simulink model "FSAC2021_V1_Running"  (R2014a)
settings: Solver=FixedStepDiscrete  StartTime=0.0  StopTime=inf  FixedStep=0.0005  RelTol=1e-3
model workspace (MAT data in the model file):
  MCOS : class17 (value not decoded)
  MCOS : class17 (value not decoded)
  MCOS : class17 (value not decoded)
  MCOS : class17 (value not decoded)
  MCOS : class17 (value not decoded)
  MCOS : class17 (value not decoded)
  MCOS : class17 (value not decoded)
  MCOS : class17 (value not decoded)
  MCOS : class17 (value not decoded)
  MCOS : class17 (value not decoded)
  MCOS : class17 (value not decoded)
  MCOS : class17 (value not decoded)
  MCOS : class17 (value not decoded)
  MCOS : class17 (value not decoded)
  MCOS : class17 (value not decoded)
  MCOS : class17 (value not decoded)
  MCOS : class17 (value not decoded)
  MCOS : class17 (value not decoded)
  MCOS : class17 (value not decoded)
  BUZZER_START = 1
  MCOS : class17 (value not decoded)
  MCOS : class17 (value not decoded)
  MCOS : class17 (value not decoded)
  MCOS : class17 (value not decoded)
  MCOS : class17 (value not decoded)
  MCOS : class17 (value not decoded)
  MCOS : class17 (value not decoded)
  MCOS : class17 (value not decoded)
  MCOS : class17 (value not decoded)
  MCOS : class17 (value not decoded)
  MCOS : class17 (value not decoded)
  MCOS : class17 (value not decoded)
  MCOS : class17 (value not decoded)
  MCOS : class17 (value not decoded)
  MCOS : class17 (value not decoded)
  MCOS : class17 (value not decoded)
  MCOS : class17 (value not decoded)
  MCOS : class17 (value not decoded)
  MCOS : class17 (value not decoded)
  MCOS : class17 (value not decoded)
  MCOS : class17 (value not decoded)
  MCOS : class17 (value not decoded)
  MCOS : class17 (value not decoded)
  MCOS : class17 (value not decoded)
  MCOS : class17 (value not decoded)
  MCOS : class17 (value not decoded)
  MCOS : class17 (value not decoded)
  MCOS : class17 (value not decoded)
  MCOS : class17 (value not decoded)
  MCOS : class17 (value not decoded)
  MCOS : class17 (value not decoded)
  MCOS : class17 (value not decoded)
  MCOS : class17 (value not decoded)
  MCOS : class17 (value not decoded)
  MCOS : class17 (value not decoded)
  MCOS : class17 (value not decoded)
  MCOS : class17 (value not decoded)
  MCOS : class17 (value not decoded)
  Brake = 11
  MCOS : class17 (value not decoded)
  MCOS : class17 (value not decoded)
  MCOS : class17 (value not decoded)
  MCOS : class17 (value not decoded)
  MCOS : class17 (value not decoded)
  MCOS : class17 (value not decoded)
  MCOS : class17 (value not decoded)
  MCOS : class17 (value not decoded)
  Sensor_Acc_b = 101.85
  Sensor_Acc_k = -0.0185
  Str_Sen_Orig_Angle = -341
  MCOS : class17 (value not decoded)
  Tire_D = 0.47
  T = 0.05
libraries: simulink x402, ec55xxlib x134
(part 9 of 17)

== system FSAC2021_V1_Running/ROUTING/TO_ACAN/DV_driving_dynamics_2/Acceleration_longitudinal ==
  Acceleration_longitudinal : Inport
  Acceleration_longitudinalABS : Abs
  Acceleration_longitudinalCOV : DataTypeConversion  OutDataTypeStr=uint8
  Acceleration_longitudinalCS : ArithShift  BitShiftNumber=-16
  Acceleration_longitudinalConS : Constant  OutDataTypeStr=single
  Acceleration_longitudinalCosR : Constant  Value=0  OutDataTypeStr=uint8
  Acceleration_longitudinalROP : RelationalOperator  Operator=<  OutDataTypeStr=boolean
  Acceleration_longitudinalRon : Rounding  Operator=round
  Acceleration_longitudinalSW : Switch  Criteria=u2 ~= 0
  Acceleration_longitudinal_1sat : Saturate  UpperLimit=65535  LowerLimit=0
  Acceleration_longitudinal_And : simulink/Logic and Bit Operations/Bitwise Operator  logicop=AND  UseBitMask=off  NumInputPorts=2  BitMask=bin2dec('11011001')  BitMaskRealWorld=Stored Integer
  Acceleration_longitudinal_And_C : Constant  Value=255  OutDataTypeStr=uint32
  Acceleration_longitudinal_Convert : DataTypeConversion  OutDataTypeStr=uint32
  Acceleration_longitudinal_D : Product  Inputs=*/
  Acceleration_longitudinal_D1 : Product  Inputs=*/
  Acceleration_longitudinal_F : Constant  Value=0.001953125  OutDataTypeStr=single
  Acceleration_longitudinal_L : simulink/Logic and Bit Operations/Bitwise Operator  logicop=AND  UseBitMask=on  BitMask=65535  BitMaskRealWorld=Stored Integer
  Acceleration_longitudinal_O : Constant  Value=0  OutDataTypeStr=single
  Acceleration_longitudinal_S : ArithShift
  Acceleration_longitudinal_sat : Saturate  UpperLimit=63.998046875  LowerLimit=-64
  Acceleration_longitudinal_st : Sum  Inputs=+-
  Acceleration_longitudinaloutput2_C : Constant  Value=256
  Acceleration_longitudinalsubcon : Sum  Inputs=+-
  BitCov : DataTypeConversion  OutDataTypeStr=uint8
  output1 : Outport
  output2 : Outport  Port=2
  wires:
  Acceleration_longitudinal/1 -> Acceleration_longitudinal_sat/1
  Acceleration_longitudinal_sat/1 -> Acceleration_longitudinal_st/1
  Acceleration_longitudinal_O/1 -> Acceleration_longitudinal_st/2
  Acceleration_longitudinal_st/1 -> Acceleration_longitudinal_D/1
  Acceleration_longitudinal_F/1 -> Acceleration_longitudinal_D/2
  Acceleration_longitudinal_D/1 -> Acceleration_longitudinalRon/1
  Acceleration_longitudinalRon/1 -> Acceleration_longitudinalROP/1, Acceleration_longitudinalABS/1, Acceleration_longitudinalSW/3
  Acceleration_longitudinalCosR/1 -> Acceleration_longitudinalROP/2
  Acceleration_longitudinalConS/1 -> Acceleration_longitudinalCS/1
  Acceleration_longitudinalCS/1 -> Acceleration_longitudinalsubcon/1
  Acceleration_longitudinalABS/1 -> Acceleration_longitudinalsubcon/2
  Acceleration_longitudinalsubcon/1 -> Acceleration_longitudinalSW/1
  Acceleration_longitudinalROP/1 -> Acceleration_longitudinalSW/2
  Acceleration_longitudinalSW/1 -> Acceleration_longitudinal_S/1
  Acceleration_longitudinal_S/1 -> Acceleration_longitudinal_1sat/1
  Acceleration_longitudinal_1sat/1 -> Acceleration_longitudinal_Convert/1
  Acceleration_longitudinal_Convert/1 -> Acceleration_longitudinal_L/1
  Acceleration_longitudinal_L/1 -> Acceleration_longitudinal_D1/1, Acceleration_longitudinal_And/1
  Acceleration_longitudinaloutput2_C/1 -> Acceleration_longitudinal_D1/2
  Acceleration_longitudinal_D1/1 -> Acceleration_longitudinalCOV/1
  Acceleration_longitudinalCOV/1 -> output2/1
  Acceleration_longitudinal_And_C/1 -> Acceleration_longitudinal_And/2
  Acceleration_longitudinal_And/1 -> BitCov/1
  BitCov/1 -> output1/1

== system FSAC2021_V1_Running/ROUTING/TO_ACAN/DV_driving_dynamics_2/Yaw_rate ==
  Yaw_rate : Inport
  BitCov : DataTypeConversion  OutDataTypeStr=uint8
  Yaw_rateABS : Abs
  Yaw_rateCOV : DataTypeConversion  OutDataTypeStr=uint8
  Yaw_rateCS : ArithShift  BitShiftNumber=-16
  Yaw_rateConS : Constant  OutDataTypeStr=single
  Yaw_rateCosR : Constant  Value=0  OutDataTypeStr=uint8
  Yaw_rateROP : RelationalOperator  Operator=<  OutDataTypeStr=boolean
  Yaw_rateRon : Rounding  Operator=round
  Yaw_rateSW : Switch  Criteria=u2 ~= 0
  Yaw_rate_1sat : Saturate  UpperLimit=65535  LowerLimit=0
  Yaw_rate_And : simulink/Logic and Bit Operations/Bitwise Operator  logicop=AND  UseBitMask=off  NumInputPorts=2  BitMask=bin2dec('11011001')  BitMaskRealWorld=Stored Integer
  Yaw_rate_And_C : Constant  Value=255  OutDataTypeStr=uint32
  Yaw_rate_Convert : DataTypeConversion  OutDataTypeStr=uint32
  Yaw_rate_D : Product  Inputs=*/
  Yaw_rate_D1 : Product  Inputs=*/
  Yaw_rate_F : Constant  Value=0.0078125  OutDataTypeStr=single
  Yaw_rate_L : simulink/Logic and Bit Operations/Bitwise Operator  logicop=AND  UseBitMask=on  BitMask=65535  BitMaskRealWorld=Stored Integer
  Yaw_rate_O : Constant  Value=0  OutDataTypeStr=single
  Yaw_rate_S : ArithShift
  Yaw_rate_sat : Saturate  UpperLimit=255.9921875  LowerLimit=-256
  Yaw_rate_st : Sum  Inputs=+-
  Yaw_rateoutput4_C : Constant  Value=256
  Yaw_ratesubcon : Sum  Inputs=+-
  output3 : Outport
  output4 : Outport  Port=2
  wires:
  Yaw_rate/1 -> Yaw_rate_sat/1
  Yaw_rate_sat/1 -> Yaw_rate_st/1
  Yaw_rate_O/1 -> Yaw_rate_st/2
  Yaw_rate_st/1 -> Yaw_rate_D/1
  Yaw_rate_F/1 -> Yaw_rate_D/2
  Yaw_rate_D/1 -> Yaw_rateRon/1
  Yaw_rateRon/1 -> Yaw_rateROP/1, Yaw_rateABS/1, Yaw_rateSW/3
  Yaw_rateCosR/1 -> Yaw_rateROP/2
  Yaw_rateConS/1 -> Yaw_rateCS/1
  Yaw_rateCS/1 -> Yaw_ratesubcon/1
  Yaw_rateABS/1 -> Yaw_ratesubcon/2
  Yaw_ratesubcon/1 -> Yaw_rateSW/1
  Yaw_rateROP/1 -> Yaw_rateSW/2
  Yaw_rateSW/1 -> Yaw_rate_S/1
  Yaw_rate_S/1 -> Yaw_rate_1sat/1
  Yaw_rate_1sat/1 -> Yaw_rate_Convert/1
  Yaw_rate_Convert/1 -> Yaw_rate_L/1
  Yaw_rate_L/1 -> Yaw_rate_D1/1, Yaw_rate_And/1
  Yaw_rateoutput4_C/1 -> Yaw_rate_D1/2
  Yaw_rate_D1/1 -> Yaw_rateCOV/1
  Yaw_rateCOV/1 -> output4/1
  Yaw_rate_And_C/1 -> Yaw_rate_And/2
  Yaw_rate_And/1 -> BitCov/1
  BitCov/1 -> output3/1

== system FSAC2021_V1_Running/ROUTING/TO_ACAN/DV_system_status/AMI_State ==
  AMI_State : Inport
  AMI_StateRon : Rounding  Operator=round
  AMI_State_1sat : Saturate  UpperLimit=7  LowerLimit=0
  AMI_State_Convert : DataTypeConversion  OutDataTypeStr=uint8
  AMI_State_Convert1 : DataTypeConversion  OutDataTypeStr=uint32
  AMI_State_D : Product  Inputs=*/
  AMI_State_F : Constant  OutDataTypeStr=single
  AMI_State_L : simulink/Logic and Bit Operations/Bitwise Operator  logicop=AND  UseBitMask=on  BitMask=7  BitMaskRealWorld=Stored Integer
  AMI_State_O : Constant  Value=0  OutDataTypeStr=single
  AMI_State_S : ArithShift
  AMI_State_sat : Saturate  UpperLimit=5  LowerLimit=0
  AMI_State_st : Sum  Inputs=+-
  output1 : Outport
  wires:
  AMI_State/1 -> AMI_State_sat/1
  AMI_State_sat/1 -> AMI_State_st/1
  AMI_State_O/1 -> AMI_State_st/2
  AMI_State_st/1 -> AMI_State_D/1
  AMI_State_F/1 -> AMI_State_D/2
  AMI_State_D/1 -> AMI_StateRon/1
  AMI_StateRon/1 -> AMI_State_S/1
  AMI_State_S/1 -> AMI_State_1sat/1
  AMI_State_1sat/1 -> AMI_State_Convert1/1
  AMI_State_Convert1/1 -> AMI_State_L/1
  AMI_State_L/1 -> AMI_State_Convert/1
  AMI_State_Convert/1 -> output1/1

== system FSAC2021_V1_Running/ROUTING/TO_ACAN/DV_system_status/ASSI_State ==
  ASSI_State : Inport
  ASSI_StateRon : Rounding  Operator=round
  ASSI_State_1sat : Saturate  UpperLimit=56  LowerLimit=0
  ASSI_State_Convert : DataTypeConversion  OutDataTypeStr=uint8
  ASSI_State_Convert1 : DataTypeConversion  OutDataTypeStr=uint32
  ASSI_State_D : Product  Inputs=*/
  ASSI_State_F : Constant  OutDataTypeStr=single
  ASSI_State_L : simulink/Logic and Bit Operations/Bitwise Operator  logicop=AND  UseBitMask=on  BitMask=56  BitMaskRealWorld=Stored Integer
  ASSI_State_O : Constant  Value=0  OutDataTypeStr=single
  ASSI_State_S : ArithShift  BitShiftNumber=-3
  ASSI_State_sat : Saturate  UpperLimit=6  LowerLimit=1
  ASSI_State_st : Sum  Inputs=+-
  output1 : Outport
  wires:
  ASSI_State/1 -> ASSI_State_sat/1
  ASSI_State_sat/1 -> ASSI_State_st/1
  ASSI_State_O/1 -> ASSI_State_st/2
  ASSI_State_st/1 -> ASSI_State_D/1
  ASSI_State_F/1 -> ASSI_State_D/2
  ASSI_State_D/1 -> ASSI_StateRon/1
  ASSI_StateRon/1 -> ASSI_State_S/1
  ASSI_State_S/1 -> ASSI_State_1sat/1
  ASSI_State_1sat/1 -> ASSI_State_Convert1/1
  ASSI_State_Convert1/1 -> ASSI_State_L/1
  ASSI_State_L/1 -> ASSI_State_Convert/1
  ASSI_State_Convert/1 -> output1/1

== system FSAC2021_V1_Running/ROUTING/TO_ACAN/DV_system_status/Cones_count_actual ==
  Cones_count_actual : Inport
  BitCov : DataTypeConversion  OutDataTypeStr=uint8
  Cones_count_actualCOV : DataTypeConversion  OutDataTypeStr=uint8
  Cones_count_actualRon : Rounding  Operator=round
  Cones_count_actual_1sat : Saturate  UpperLimit=32640  LowerLimit=0
  Cones_count_actual_And : simulink/Logic and Bit Operations/Bitwise Operator  logicop=AND  UseBitMask=off  NumInputPorts=2  BitMask=bin2dec('11011001')  BitMaskRealWorld=Stored Integer
  Cones_count_actual_And_C : Constant  Value=255  OutDataTypeStr=uint32
  Cones_count_actual_Convert : DataTypeConversion  OutDataTypeStr=uint32
  Cones_count_actual_D : Product  Inputs=*/
  Cones_count_actual_D1 : Product  Inputs=*/
  Cones_count_actual_F : Constant  OutDataTypeStr=single
  Cones_count_actual_L : simulink/Logic and Bit Operations/Bitwise Operator  logicop=AND  UseBitMask=on  BitMask=32640  BitMaskRealWorld=Stored Integer
  Cones_count_actual_O : Constant  Value=0  OutDataTypeStr=single
  Cones_count_actual_S : ArithShift  BitShiftNumber=-7
  Cones_count_actual_sat : Saturate  UpperLimit=255  LowerLimit=0
  Cones_count_actual_st : Sum  Inputs=+-
  Cones_count_actualoutput3_C : Constant  Value=256
  output2 : Outport
  output3 : Outport  Port=2
  wires:
  Cones_count_actual/1 -> Cones_count_actual_sat/1
  Cones_count_actual_sat/1 -> Cones_count_actual_st/1
  Cones_count_actual_O/1 -> Cones_count_actual_st/2
  Cones_count_actual_st/1 -> Cones_count_actual_D/1
  Cones_count_actual_F/1 -> Cones_count_actual_D/2
  Cones_count_actual_D/1 -> Cones_count_actualRon/1
  Cones_count_actualRon/1 -> Cones_count_actual_S/1
  Cones_count_actual_S/1 -> Cones_count_actual_1sat/1
  Cones_count_actual_1sat/1 -> Cones_count_actual_Convert/1
  Cones_count_actual_Convert/1 -> Cones_count_actual_L/1
  Cones_count_actual_L/1 -> Cones_count_actual_D1/1, Cones_count_actual_And/1
  Cones_count_actualoutput3_C/1 -> Cones_count_actual_D1/2
  Cones_count_actual_D1/1 -> Cones_count_actualCOV/1
  Cones_count_actualCOV/1 -> output3/1
  Cones_count_actual_And_C/1 -> Cones_count_actual_And/2
  Cones_count_actual_And/1 -> BitCov/1
  BitCov/1 -> output2/1

== system FSAC2021_V1_Running/ROUTING/TO_ACAN/DV_system_status/Cones_count_all ==
  Cones_count_all : Inport
  Cones_count_allBitCov : DataTypeConversion  OutDataTypeStr=uint32
  Cones_count_allBitCov1 : DataTypeConversion  OutDataTypeStr=uint8
  Cones_count_allCOV : DataTypeConversion  OutDataTypeStr=uint8
  Cones_count_allCOV1 : DataTypeConversion  OutDataTypeStr=uint8
  Cones_count_allRon : Rounding  Operator=round
  Cones_count_all_1sat : Saturate  UpperLimit=16777088  LowerLimit=0
  Cones_count_all_And : simulink/Logic and Bit Operations/Bitwise Operator  logicop=AND  UseBitMask=off  NumInputPorts=2  BitMask=bin2dec('11011001')  BitMaskRealWorld=Stored Integer
  Cones_count_all_And1 : simulink/Logic and Bit Operations/Bitwise Operator  logicop=AND  UseBitMask=off  NumInputPorts=2  BitMask=bin2dec('11011001')  BitMaskRealWorld=Stored Integer
  Cones_count_all_And1_C : Constant  Value=255  OutDataTypeStr=uint32
  Cones_count_all_And_C : Constant  Value=65535
  Cones_count_all_Convert : DataTypeConversion  OutDataTypeStr=uint32
  Cones_count_all_D : Product  Inputs=*/
  Cones_count_all_D1 : Product  Inputs=*/
  Cones_count_all_D2 : Product  Inputs=*/
  Cones_count_all_F : Constant  OutDataTypeStr=single
  Cones_count_all_L : simulink/Logic and Bit Operations/Bitwise Operator  logicop=AND  UseBitMask=on  BitMask=16777088  BitMaskRealWorld=Stored Integer
  Cones_count_all_O : Constant  Value=0  OutDataTypeStr=single
  Cones_count_all_S : ArithShift  BitShiftNumber=-7
  Cones_count_all_sat : Saturate  UpperLimit=131071  LowerLimit=0
  Cones_count_all_st : Sum  Inputs=+-
  Cones_count_alloutput4_C : Constant  Value=256
  Cones_count_alloutput5_C : Constant  Value=65536
  output3 : Outport
  output4 : Outport  Port=2
  output5 : Outport  Port=3
  wires:
  Cones_count_all/1 -> Cones_count_all_sat/1
  Cones_count_all_sat/1 -> Cones_count_all_st/1
  Cones_count_all_O/1 -> Cones_count_all_st/2
  Cones_count_all_st/1 -> Cones_count_all_D/1
  Cones_count_all_F/1 -> Cones_count_all_D/2
  Cones_count_all_D/1 -> Cones_count_allRon/1
  Cones_count_allRon/1 -> Cones_count_all_S/1
  Cones_count_all_S/1 -> Cones_count_all_1sat/1
  Cones_count_all_1sat/1 -> Cones_count_all_Convert/1
  Cones_count_all_Convert/1 -> Cones_count_all_L/1
  Cones_count_all_L/1 -> Cones_count_all_And/1, Cones_count_all_And1/1, Cones_count_all_D1/1
  Cones_count_alloutput5_C/1 -> Cones_count_all_D1/2
  Cones_count_all_D1/1 -> Cones_count_allCOV/1
  Cones_count_allCOV/1 -> output5/1
  Cones_count_all_And_C/1 -> Cones_count_allBitCov/1
  Cones_count_allBitCov/1 -> Cones_count_all_And/2
  Cones_count_all_And/1 -> Cones_count_all_D2/1
  Cones_count_alloutput4_C/1 -> Cones_count_all_D2/2
  Cones_count_all_D2/1 -> Cones_count_allCOV1/1
  Cones_count_allCOV1/1 -> output4/1
  Cones_count_all_And1_C/1 -> Cones_count_all_And1/2
  Cones_count_all_And1/1 -> Cones_count_allBitCov1/1
  Cones_count_allBitCov1/1 -> output3/1

== system FSAC2021_V1_Running/ROUTING/TO_ACAN/DV_system_status/EBS_State ==
  EBS_State : Inport
  EBS_StateRon : Rounding  Operator=round
  EBS_State_1sat : Saturate  UpperLimit=192  LowerLimit=0
  EBS_State_Convert : DataTypeConversion  OutDataTypeStr=uint8
  EBS_State_Convert1 : DataTypeConversion  OutDataTypeStr=uint32
  EBS_State_D : Product  Inputs=*/
  EBS_State_F : Constant  OutDataTypeStr=single
  EBS_State_L : simulink/Logic and Bit Operations/Bitwise Operator  logicop=AND  UseBitMask=on  BitMask=192  BitMaskRealWorld=Stored Integer
  EBS_State_O : Constant  Value=0  OutDataTypeStr=single
  EBS_State_S : ArithShift  BitShiftNumber=-6
  EBS_State_sat : Saturate  UpperLimit=3  LowerLimit=1
  EBS_State_st : Sum  Inputs=+-
  output1 : Outport
  wires:
  EBS_State/1 -> EBS_State_sat/1
  EBS_State_sat/1 -> EBS_State_st/1
  EBS_State_O/1 -> EBS_State_st/2
  EBS_State_st/1 -> EBS_State_D/1
  EBS_State_F/1 -> EBS_State_D/2
  EBS_State_D/1 -> EBS_StateRon/1
  EBS_StateRon/1 -> EBS_State_S/1
  EBS_State_S/1 -> EBS_State_1sat/1
  EBS_State_1sat/1 -> EBS_State_Convert1/1
  EBS_State_Convert1/1 -> EBS_State_L/1
  EBS_State_L/1 -> EBS_State_Convert/1
  EBS_State_Convert/1 -> output1/1

== system FSAC2021_V1_Running/ROUTING/TO_ACAN/DV_system_status/Lap_counter ==
  Lap_counter : Inport
  Lap_counterRon : Rounding  Operator=round
  Lap_counter_1sat : Saturate  UpperLimit=120  LowerLimit=0
  Lap_counter_Convert : DataTypeConversion  OutDataTypeStr=uint8
  Lap_counter_Convert1 : DataTypeConversion  OutDataTypeStr=uint32
  Lap_counter_D : Product  Inputs=*/
  Lap_counter_F : Constant  OutDataTypeStr=single
  Lap_counter_L : simulink/Logic and Bit Operations/Bitwise Operator  logicop=AND  UseBitMask=on  BitMask=120  BitMaskRealWorld=Stored Integer
  Lap_counter_O : Constant  Value=0  OutDataTypeStr=single
  Lap_counter_S : ArithShift  BitShiftNumber=-3
  Lap_counter_sat : Saturate  UpperLimit=15  LowerLimit=0
  Lap_counter_st : Sum  Inputs=+-
  output2 : Outport
  wires:
  Lap_counter/1 -> Lap_counter_sat/1
  Lap_counter_sat/1 -> Lap_counter_st/1
  Lap_counter_O/1 -> Lap_counter_st/2
  Lap_counter_st/1 -> Lap_counter_D/1
  Lap_counter_F/1 -> Lap_counter_D/2
  Lap_counter_D/1 -> Lap_counterRon/1
  Lap_counterRon/1 -> Lap_counter_S/1
  Lap_counter_S/1 -> Lap_counter_1sat/1
  Lap_counter_1sat/1 -> Lap_counter_Convert1/1
  Lap_counter_Convert1/1 -> Lap_counter_L/1
  Lap_counter_L/1 -> Lap_counter_Convert/1
  Lap_counter_Convert/1 -> output2/1

== system FSAC2021_V1_Running/ROUTING/TO_ACAN/DV_system_status/Service_brake_state ==
  Service_brake_state : Inport
  Service_brake_stateRon : Rounding  Operator=round
  Service_brake_state_1sat : Saturate  UpperLimit=6  LowerLimit=0
  Service_brake_state_Convert : DataTypeConversion  OutDataTypeStr=uint8
  Service_brake_state_Convert1 : DataTypeConversion  OutDataTypeStr=uint32
  Service_brake_state_D : Product  Inputs=*/
  Service_brake_state_F : Constant  OutDataTypeStr=single
  Service_brake_state_L : simulink/Logic and Bit Operations/Bitwise Operator  logicop=AND  UseBitMask=on  BitMask=6  BitMaskRealWorld=Stored Integer
  Service_brake_state_O : Constant  Value=0  OutDataTypeStr=single
  Service_brake_state_S : ArithShift  BitShiftNumber=-1
  Service_brake_state_sat : Saturate  UpperLimit=3  LowerLimit=1
  Service_brake_state_st : Sum  Inputs=+-
  output2 : Outport
  wires:
  Service_brake_state/1 -> Service_brake_state_sat/1
  Service_brake_state_sat/1 -> Service_brake_state_st/1
  Service_brake_state_O/1 -> Service_brake_state_st/2
  Service_brake_state_st/1 -> Service_brake_state_D/1
  Service_brake_state_F/1 -> Service_brake_state_D/2
  Service_brake_state_D/1 -> Service_brake_stateRon/1
  Service_brake_stateRon/1 -> Service_brake_state_S/1
  Service_brake_state_S/1 -> Service_brake_state_1sat/1
  Service_brake_state_1sat/1 -> Service_brake_state_Convert1/1
  Service_brake_state_Convert1/1 -> Service_brake_state_L/1
  Service_brake_state_L/1 -> Service_brake_state_Convert/1
  Service_brake_state_Convert/1 -> output2/1

== system FSAC2021_V1_Running/ROUTING/TO_ACAN/DV_system_status/Steering_state ==
  Steering_state : Inport
  Steering_stateRon : Rounding  Operator=round
  Steering_state_1sat : Saturate  UpperLimit=1  LowerLimit=0
  Steering_state_Convert : DataTypeConversion  OutDataTypeStr=uint8
  Steering_state_Convert1 : DataTypeConversion  OutDataTypeStr=uint32
  Steering_state_D : Product  Inputs=*/
  Steering_state_F : Constant  OutDataTypeStr=single
  Steering_state_L : simulink/Logic and Bit Operations/Bitwise Operator  logicop=AND  UseBitMask=on  BitMask=1  BitMaskRealWorld=Stored Integer
  Steering_state_O : Constant  Value=0  OutDataTypeStr=single
  Steering_state_S : ArithShift
  Steering_state_sat : Saturate  UpperLimit=1  LowerLimit=0
  Steering_state_st : Sum  Inputs=+-
  output2 : Outport
  wires:
  Steering_state/1 -> Steering_state_sat/1
  Steering_state_sat/1 -> Steering_state_st/1
  Steering_state_O/1 -> Steering_state_st/2
  Steering_state_st/1 -> Steering_state_D/1
  Steering_state_F/1 -> Steering_state_D/2
  Steering_state_D/1 -> Steering_stateRon/1
  Steering_stateRon/1 -> Steering_state_S/1
  Steering_state_S/1 -> Steering_state_1sat/1
  Steering_state_1sat/1 -> Steering_state_Convert1/1
  Steering_state_Convert1/1 -> Steering_state_L/1
  Steering_state_L/1 -> Steering_state_Convert/1
  Steering_state_Convert/1 -> output2/1

== system FSAC2021_V1_Running/ROUTING/TO_DCAN/Subsystem/DIAG_BCU ==
  Brake_sensor6_sts_in : Inport
  Brake_sensor5_sts_in : Inport  Port=2
  Brake_sensor4_sts_in : Inport  Port=3
  Brake_sensor3_sts_in : Inport  Port=4
  Brake_sensor2_sts_in : Inport  Port=5
  Brake_sensor1_sts_in : Inport  Port=6
  Brake_reg_rw_fault_flag_in : Inport  Port=7
  Brake_overheat_prtct_sts_in : Inport  Port=8
  Brake_overcurrt_prtct_sts_in : Inport  Port=9
  Brake_mtr_stop_flag_in : Inport  Port=10
  Brake_mtr_origin_flag_in : Inport  Port=11
  Brake_mtr_enable_flag_in : Inport  Port=12
  Brake_lowvolt_prtct_sts_in : Inport  Port=13
  Brake_encoder_fault_sts_in : Inport  Port=14
  Brake_Current_Position_in : Inport  Port=15
  Brake_cmd_fault_flag_in : Inport  Port=16
  Brake_0rigin_End_flag_in : Inport  Port=17
  Brake_0rigin_End_flag : Subsystem
  Brake_Current_Position : Subsystem
  Brake_cmd_fault_flag : Subsystem
  Brake_encoder_fault_sts : Subsystem
  Brake_lowvolt_prtct_sts : Subsystem
  Brake_mtr_enable_flag : Subsystem
  Brake_mtr_origin_flag : Subsystem
  Brake_mtr_stop_flag : Subsystem
  Brake_overcurrt_prtct_sts : Subsystem
  Brake_overheat_prtct_sts : Subsystem
  Brake_reg_rw_fault_flag : Subsystem
  Brake_sensor1_sts : Subsystem
  Brake_sensor2_sts : Subsystem
  Brake_sensor3_sts : Subsystem
  Brake_sensor4_sts : Subsystem
  Brake_sensor5_sts : Subsystem
  Brake_sensor6_sts : Subsystem
  Conv{1..4} (4 alike) : DataTypeConversion
  DIAG_BCU_mux : Mux
  or3 : simulink/Logic and Bit Operations/Bitwise Operator  logicop=OR  UseBitMask=off  NumInputPorts=8  BitMask=bin2dec('11011001')  BitMaskRealWorld=Stored Integer
  or4 : simulink/Logic and Bit Operations/Bitwise Operator  logicop=OR  UseBitMask=off  NumInputPorts=8  BitMask=bin2dec('11011001')  BitMaskRealWorld=Stored Integer
  output : Outport
  wires:
  DIAG_BCU_mux/1 -> output/1
  Brake_sensor6_sts/1(output3) -> or3/1
  Brake_sensor5_sts/1(output3) -> or3/2
  Brake_sensor4_sts/1(output3) -> or3/3
  Brake_sensor3_sts/1(output3) -> or3/4
  Brake_sensor2_sts/1(output3) -> or3/5
  Brake_sensor1_sts/1(output3) -> or3/6
  Brake_reg_rw_fault_flag/1(output4) -> or4/7
  Brake_overheat_prtct_sts/1(output4) -> or4/8
  Brake_overcurrt_prtct_sts/1(output4) -> or4/1
  Brake_mtr_stop_flag/1(output3) -> or3/7
  Brake_mtr_origin_flag/1(output3) -> or3/8
  Brake_mtr_enable_flag/1(output4) -> or4/2
  Brake_lowvolt_prtct_sts/1(output4) -> or4/3
  Brake_encoder_fault_sts/1(output4) -> or4/4
  Brake_cmd_fault_flag/1(output4) -> or4/5
  Brake_0rigin_End_flag/1(output4) -> or4/6
  Brake_Current_Position/1(output1) -> Conv1/1
  Conv1/1 -> DIAG_BCU_mux/1
  Brake_Current_Position/2(output2) -> Conv2/1
  Conv2/1 -> DIAG_BCU_mux/2
  or3/1 -> Conv3/1
  Conv3/1 -> DIAG_BCU_mux/3
  or4/1 -> Conv4/1
  Conv4/1 -> DIAG_BCU_mux/4
  Brake_sensor6_sts_in/1 -> Brake_sensor6_sts/1(Brake_sensor6_sts)
  Brake_sensor5_sts_in/1 -> Brake_sensor5_sts/1(Brake_sensor5_sts)
  Brake_sensor4_sts_in/1 -> Brake_sensor4_sts/1(Brake_sensor4_sts)
  Brake_sensor3_sts_in/1 -> Brake_sensor3_sts/1(Brake_sensor3_sts)
  Brake_sensor2_sts_in/1 -> Brake_sensor2_sts/1(Brake_sensor2_sts)
  Brake_sensor1_sts_in/1 -> Brake_sensor1_sts/1(Brake_sensor1_sts)
  Brake_reg_rw_fault_flag_in/1 -> Brake_reg_rw_fault_flag/1(Brake_reg_rw_fault_flag)
  Brake_overheat_prtct_sts_in/1 -> Brake_overheat_prtct_sts/1(Brake_overheat_prtct_sts)
  Brake_overcurrt_prtct_sts_in/1 -> Brake_overcurrt_prtct_sts/1(Brake_overcurrt_prtct_sts)
  Brake_mtr_stop_flag_in/1 -> Brake_mtr_stop_flag/1(Brake_mtr_stop_flag)
  Brake_mtr_origin_flag_in/1 -> Brake_mtr_origin_flag/1(Brake_mtr_origin_flag)
  Brake_mtr_enable_flag_in/1 -> Brake_mtr_enable_flag/1(Brake_mtr_enable_flag)
  Brake_lowvolt_prtct_sts_in/1 -> Brake_lowvolt_prtct_sts/1(Brake_lowvolt_prtct_sts)
  Brake_encoder_fault_sts_in/1 -> Brake_encoder_fault_sts/1(Brake_encoder_fault_sts)
  Brake_Current_Position_in/1 -> Brake_Current_Position/1(Brake_Current_Position)
  Brake_cmd_fault_flag_in/1 -> Brake_cmd_fault_flag/1(Brake_cmd_fault_flag)
  Brake_0rigin_End_flag_in/1 -> Brake_0rigin_End_flag/1(Brake_0rigin_End_flag)

== system FSAC2021_V1_Running/ROUTING/TO_DCAN/Subsystem/DIAG_BMS_ALARM_RELAY ==
  PreRlyStr_in : Inport
  PosRlyStr_in : Inport  Port=2
  OnChrRlyStr_in : Inport  Port=3
  NegRlyStr_in : Inport  Port=4
  ALM_PRECHRG_FAIL_in : Inport  Port=5
  ALM_LEAK_OC_in : Inport  Port=6
  ALM_HVREL_FAIL_in : Inport  Port=7
  ALM_HALL_BREAK_in : Inport  Port=8
  ALM_DSCH_OCT_in : Inport  Port=9
  ALM_DSCH_OCS_in : Inport  Port=10
  ALM_CHRG_OCT_in : Inport  Port=11
  ALM_CHRG_OCS_in : Inport  Port=12
  ALM_BSU_OFFLINE_in : Inport  Port=13
  ALM_BSU_FAULT_in : Inport  Port=14
  ALM_BMU_FAIL_in : Inport  Port=15
  ALM_BATT_UC_in : Inport  Port=16
  ALM_BATT_OC_in : Inport  Port=17
  ALM_AUX_FAIL_in : Inport  Port=18
  ALM_BATT_UV_in : Inport  Port=19
  ALM_BATT_OV_in : Inport  Port=20
  ALM_BATT_DT_in : Inport  Port=21
  ALM_BATT_DV_in : Inport  Port=22
  ALM_CELL_TBK_in : Inport  Port=23
  ALM_CELL_IBK_in : Inport  Port=24
  ALM_CELL_UT_in : Inport  Port=25
  ALM_CELL_OT_in : Inport  Port=26
  ALM_CELL_UV_in : Inport  Port=27
  ALM_CELL_OV_in : Inport  Port=28
  ALM_AUX_FAIL : Subsystem
  ALM_BATT_DT : Subsystem
  ALM_BATT_DV : Subsystem
  ALM_BATT_OC : Subsystem
  ALM_BATT_OV : Subsystem
  ALM_BATT_UC : Subsystem
  ALM_BATT_UV : Subsystem
  ALM_BMU_FAIL : Subsystem
  ALM_BSU_FAULT : Subsystem
  ALM_BSU_OFFLINE : Subsystem
  ALM_CELL_IBK : Subsystem
  ALM_CELL_OT : Subsystem
  ALM_CELL_OV : Subsystem
  ALM_CELL_TBK : Subsystem
  ALM_CELL_UT : Subsystem
  ALM_CELL_UV : Subsystem
  ALM_CHRG_OCS : Subsystem
  ALM_CHRG_OCT : Subsystem
  ALM_DSCH_OCS : Subsystem
  ALM_DSCH_OCT : Subsystem
  ALM_HALL_BREAK : Subsystem
  ALM_HVREL_FAIL : Subsystem
  ALM_LEAK_OC : Subsystem
  ALM_PRECHRG_FAIL : Subsystem
  Conv{1..4} (4 alike) : DataTypeConversion
  DIAG_BMS_ALARM_RELAY_mux : Mux
  NegRlyStr : Subsystem
  OnChrRlyStr : Subsystem
  PosRlyStr : Subsystem
  PreRlyStr : Subsystem
  or1 : simulink/Logic and Bit Operations/Bitwise Operator  logicop=OR  UseBitMask=off  NumInputPorts=8  BitMask=bin2dec('11011001')  BitMaskRealWorld=Stored Integer
  or2 : simulink/Logic and Bit Operations/Bitwise Operator  logicop=OR  UseBitMask=off  NumInputPorts=8  BitMask=bin2dec('11011001')  BitMaskRealWorld=Stored Integer
  or3 : simulink/Logic and Bit Operations/Bitwise Operator  logicop=OR  UseBitMask=off  NumInputPorts=8  BitMask=bin2dec('11011001')  BitMaskRealWorld=Stored Integer
  or4 : simulink/Logic and Bit Operations/Bitwise Operator  logicop=OR  UseBitMask=off  NumInputPorts=4  BitMask=bin2dec('11011001')  BitMaskRealWorld=Stored Integer
  output : Outport
  wires:
  DIAG_BMS_ALARM_RELAY_mux/1 -> output/1
  PreRlyStr/1(output4) -> or4/1
  PosRlyStr/1(output4) -> or4/2
  OnChrRlyStr/1(output4) -> or4/3
  NegRlyStr/1(output4) -> or4/4
  ALM_PRECHRG_FAIL/1(output3) -> or3/1
  ALM_LEAK_OC/1(output3) -> or3/2
  ALM_HVREL_FAIL/1(output3) -> or3/3
  ALM_HALL_BREAK/1(output3) -> or3/4
  ALM_DSCH_OCT/1(output2) -> or2/1
  ALM_DSCH_OCS/1(output2) -> or2/2
  ALM_CHRG_OCT/1(output2) -> or2/3
  ALM_CHRG_OCS/1(output2) -> or2/4
  ALM_BSU_OFFLINE/1(output3) -> or3/5
  ALM_BSU_FAULT/1(output3) -> or3/7
  ALM_BMU_FAIL/1(output3) -> or3/6
  ALM_BATT_UC/1(output2) -> or2/5
  ALM_BATT_OC/1(output2) -> or2/6
  ALM_AUX_FAIL/1(output3) -> or3/8
  ALM_BATT_UV/1(output2) -> or2/7
  ALM_BATT_OV/1(output2) -> or2/8
  ALM_BATT_DT/1(output1) -> or1/1
  ALM_BATT_DV/1(output1) -> or1/2
  ALM_CELL_TBK/1(output1) -> or1/3
  ALM_CELL_IBK/1(output1) -> or1/4
  ALM_CELL_UT/1(output1) -> or1/5
  ALM_CELL_OT/1(output1) -> or1/6
  ALM_CELL_UV/1(output1) -> or1/7
  ALM_CELL_OV/1(output1) -> or1/8
  or1/1 -> Conv1/1
  Conv1/1 -> DIAG_BMS_ALARM_RELAY_mux/1
  or2/1 -> Conv2/1
  Conv2/1 -> DIAG_BMS_ALARM_RELAY_mux/2
  or3/1 -> Conv3/1
  Conv3/1 -> DIAG_BMS_ALARM_RELAY_mux/3
  or4/1 -> Conv4/1
  Conv4/1 -> DIAG_BMS_ALARM_RELAY_mux/4
  PreRlyStr_in/1 -> PreRlyStr/1(PreRlyStr)
  PosRlyStr_in/1 -> PosRlyStr/1(PosRlyStr)
  OnChrRlyStr_in/1 -> OnChrRlyStr/1(OnChrRlyStr)
  NegRlyStr_in/1 -> NegRlyStr/1(NegRlyStr)
  ALM_PRECHRG_FAIL_in/1 -> ALM_PRECHRG_FAIL/1(ALM_PRECHRG_FAIL)
  ALM_LEAK_OC_in/1 -> ALM_LEAK_OC/1(ALM_LEAK_OC)
  ALM_HVREL_FAIL_in/1 -> ALM_HVREL_FAIL/1(ALM_HVREL_FAIL)
  ALM_HALL_BREAK_in/1 -> ALM_HALL_BREAK/1(ALM_HALL_BREAK)
  ALM_DSCH_OCT_in/1 -> ALM_DSCH_OCT/1(ALM_DSCH_OCT)
  ALM_DSCH_OCS_in/1 -> ALM_DSCH_OCS/1(ALM_DSCH_OCS)
  ALM_CHRG_OCT_in/1 -> ALM_CHRG_OCT/1(ALM_CHRG_OCT)
  ALM_CHRG_OCS_in/1 -> ALM_CHRG_OCS/1(ALM_CHRG_OCS)
  ALM_BSU_OFFLINE_in/1 -> ALM_BSU_OFFLINE/1(ALM_BSU_OFFLINE)
  ALM_BSU_FAULT_in/1 -> ALM_BSU_FAULT/1(ALM_BSU_FAULT)
  ALM_BMU_FAIL_in/1 -> ALM_BMU_FAIL/1(ALM_BMU_FAIL)
  ALM_BATT_UC_in/1 -> ALM_BATT_UC/1(ALM_BATT_UC)
  ALM_BATT_OC_in/1 -> ALM_BATT_OC/1(ALM_BATT_OC)
  ALM_AUX_FAIL_in/1 -> ALM_AUX_FAIL/1(ALM_AUX_FAIL)
  ALM_BATT_UV_in/1 -> ALM_BATT_UV/1(ALM_BATT_UV)
  ALM_BATT_OV_in/1 -> ALM_BATT_OV/1(ALM_BATT_OV)
  ALM_BATT_DT_in/1 -> ALM_BATT_DT/1(ALM_BATT_DT)
  ALM_BATT_DV_in/1 -> ALM_BATT_DV/1(ALM_BATT_DV)
  ALM_CELL_TBK_in/1 -> ALM_CELL_TBK/1(ALM_CELL_TBK)
  ALM_CELL_IBK_in/1 -> ALM_CELL_IBK/1(ALM_CELL_IBK)
  ALM_CELL_UT_in/1 -> ALM_CELL_UT/1(ALM_CELL_UT)
  ALM_CELL_OT_in/1 -> ALM_CELL_OT/1(ALM_CELL_OT)
  ALM_CELL_UV_in/1 -> ALM_CELL_UV/1(ALM_CELL_UV)
  ALM_CELL_OV_in/1 -> ALM_CELL_OV/1(ALM_CELL_OV)

== system FSAC2021_V1_Running/ROUTING/TO_DCAN/Subsystem/DIAG_BMS_INFO ==
  BatLife_in : Inport
  BatAlmLv_in : Inport  Port=2
  BatState_in : Inport  Port=3
  BatSoh_in : Inport  Port=4
  BatSoc_in : Inport  Port=5
  BatCurrent_in : Inport  Port=6
  BatVoltage_in : Inport  Port=7
  BatAlmLv : Subsystem
  BatCurrent : Subsystem
  BatLife : Subsystem
  BatSoc : Subsystem
  BatSoh : Subsystem
  BatState : Subsystem
  BatVoltage : Subsystem
  Conv{1..8} (8 alike) : DataTypeConversion
  DIAG_BMS_INFO_mux : Mux  Inputs=8
  or7 : simulink/Logic and Bit Operations/Bitwise Operator  logicop=OR  UseBitMask=off  NumInputPorts=2  BitMask=bin2dec('11011001')  BitMaskRealWorld=Stored Integer
  output : Outport
  wires:
  DIAG_BMS_INFO_mux/1 -> output/1
  BatAlmLv/1(output7) -> or7/2
  BatState/1(output7) -> or7/1
  BatVoltage/1(output1) -> Conv1/1
  Conv1/1 -> DIAG_BMS_INFO_mux/1
  BatVoltage/2(output2) -> Conv2/1
  Conv2/1 -> DIAG_BMS_INFO_mux/2
  BatCurrent/1(output3) -> Conv3/1
  Conv3/1 -> DIAG_BMS_INFO_mux/3
  BatCurrent/2(output4) -> Conv4/1
  Conv4/1 -> DIAG_BMS_INFO_mux/4
  BatSoc/1(output5) -> Conv5/1
  Conv5/1 -> DIAG_BMS_INFO_mux/5
  BatSoh/1(output6) -> Conv6/1
  Conv6/1 -> DIAG_BMS_INFO_mux/6
  or7/1 -> Conv7/1
  Conv7/1 -> DIAG_BMS_INFO_mux/7
  BatLife/1(output8) -> Conv8/1
  Conv8/1 -> DIAG_BMS_INFO_mux/8
  BatLife_in/1 -> BatLife/1(BatLife)
  BatAlmLv_in/1 -> BatAlmLv/1(BatAlmLv)
  BatState_in/1 -> BatState/1(BatState)
  BatSoh_in/1 -> BatSoh/1(BatSoh)
  BatSoc_in/1 -> BatSoc/1(BatSoc)
  BatCurrent_in/1 -> BatCurrent/1(BatCurrent)
  BatVoltage_in/1 -> BatVoltage/1(BatVoltage)

== system FSAC2021_V1_Running/ROUTING/TO_DCAN/Subsystem/DIAG_BMS_MAXT ==
  MinTempNo_in : Inport
  MaxTempNo_in : Inport  Port=2
  MinTemp_in : Inport  Port=3
  MaxTemp_in : Inport  Port=4
  Conv{1..4} (4 alike) : DataTypeConversion
  DIAG_BMS_MAXT_mux : Mux
  MaxTemp : Subsystem
  MaxTempNo : Subsystem
  MinTemp : Subsystem
  MinTempNo : Subsystem
  output : Outport
  wires:
  DIAG_BMS_MAXT_mux/1 -> output/1
  MinTemp/1(output2) -> Conv2/1
  MaxTemp/1(output1) -> Conv1/1
  Conv1/1 -> DIAG_BMS_MAXT_mux/1
  Conv2/1 -> DIAG_BMS_MAXT_mux/2
  MaxTempNo/1(output3) -> Conv3/1
  Conv3/1 -> DIAG_BMS_MAXT_mux/3
  MinTempNo/1(output4) -> Conv4/1
  Conv4/1 -> DIAG_BMS_MAXT_mux/4
  MinTempNo_in/1 -> MinTempNo/1(MinTempNo)
  MaxTempNo_in/1 -> MaxTempNo/1(MaxTempNo)
  MinTemp_in/1 -> MinTemp/1(MinTemp)
  MaxTemp_in/1 -> MaxTemp/1(MaxTemp)

== system FSAC2021_V1_Running/ROUTING/TO_DCAN/Subsystem/DIAG_BMS_MAXV ==
  MaxCellVoltNo_in : Inport
  MinCellVoltNo_in : Inport  Port=2
  MinCellVolt_in : Inport  Port=3
  MaxCellVolt_in : Inport  Port=4
  Conv{1..6} (6 alike) : DataTypeConversion
  DIAG_BMS_MAXV_mux : Mux  Inputs=6
  MaxCellVolt : Subsystem
  MaxCellVoltNo : Subsystem
  MinCellVolt : Subsystem
  MinCellVoltNo : Subsystem
  output : Outport
  wires:
  DIAG_BMS_MAXV_mux/1 -> output/1
  MaxCellVolt/1(output1) -> Conv1/1
  Conv1/1 -> DIAG_BMS_MAXV_mux/1
  MaxCellVolt/2(output2) -> Conv2/1
  Conv2/1 -> DIAG_BMS_MAXV_mux/2
  MinCellVolt/1(output3) -> Conv3/1
  Conv3/1 -> DIAG_BMS_MAXV_mux/3
  MinCellVolt/2(output4) -> Conv4/1
  Conv4/1 -> DIAG_BMS_MAXV_mux/4
  MinCellVoltNo/1(output5) -> Conv5/1
  Conv5/1 -> DIAG_BMS_MAXV_mux/5
  MaxCellVoltNo/1(output6) -> Conv6/1
  Conv6/1 -> DIAG_BMS_MAXV_mux/6
  MaxCellVoltNo_in/1 -> MaxCellVoltNo/1(MaxCellVoltNo)
  MinCellVoltNo_in/1 -> MinCellVoltNo/1(MinCellVoltNo)
  MinCellVolt_in/1 -> MinCellVolt/1(MinCellVolt)
  MaxCellVolt_in/1 -> MaxCellVolt/1(MaxCellVolt)

== system FSAC2021_V1_Running/ROUTING/TO_DCAN/Subsystem/DIAG_RES_INFO ==
  RES_Steering_in : Inport
  RES_Return_INFO_in : Inport  Port=2
  RES_GO_in : Inport  Port=3
  RES_EBS_in : Inport  Port=4
  RES_Brake_in : Inport  Port=5
  RES_ACC_in : Inport  Port=6
  Conv{1..8} (8 alike) : DataTypeConversion
  DIAG_RES_INFO_DLC : Constant  Value=4  OutDataTypeStr=uint8
  DIAG_RES_INFO_DLC_Out : Terminator
  DIAG_RES_INFO_ID : Constant  Value=1825  OutDataTypeStr=single
  DIAG_RES_INFO_ID_Out : Terminator
  DIAG_RES_INFO_mux : Mux  Inputs=8
  RES_ACC : Subsystem
  RES_Brake : Subsystem
  RES_EBS : Subsystem
  RES_GO : Subsystem
  RES_Return_INFO : Subsystem
  RES_Steering : Subsystem
  or{1..8} (8 alike) : simulink/Logic and Bit Operations/Bitwise Operator  logicop=OR  UseBitMask=off  NumInputPorts=6  BitMask=bin2dec('11011001')  BitMaskRealWorld=Stored Integer
  output : Outport
  wires:
  DIAG_RES_INFO_mux/1 -> output/1
  RES_Steering/1(output1) -> or1/1
  RES_Steering/2(output2) -> or2/1
  RES_Steering/3(output3) -> or3/1
  RES_Steering/4(output4) -> or4/1
  RES_Steering/5(output5) -> or5/1
  RES_Steering/6(output6) -> or6/1
  RES_Steering/7(output7) -> or7/1
  RES_Steering/8(output8) -> or8/1
  RES_Return_INFO/1(output1) -> or1/2
  RES_Return_INFO/2(output2) -> or2/2
  RES_Return_INFO/3(output3) -> or3/2
  RES_Return_INFO/4(output4) -> or4/2
  RES_Return_INFO/5(output5) -> or5/2
  RES_Return_INFO/6(output6) -> or6/2
  RES_Return_INFO/7(output7) -> or7/2
  RES_Return_INFO/8(output8) -> or8/2
  RES_GO/1(output1) -> or1/3
  RES_GO/2(output2) -> or2/3
  RES_GO/3(output3) -> or3/3
  RES_GO/4(output4) -> or4/3
  RES_GO/5(output5) -> or5/3
  RES_GO/6(output6) -> or6/3
  RES_GO/7(output7) -> or7/3
  RES_GO/8(output8) -> or8/3
  RES_EBS/1(output1) -> or1/4
  RES_EBS/2(output2) -> or2/4
  RES_EBS/3(output3) -> or3/4
  RES_EBS/4(output4) -> or4/4
  RES_EBS/5(output5) -> or5/4
  RES_EBS/6(output6) -> or6/4
  RES_EBS/7(output7) -> or7/4
  RES_EBS/8(output8) -> or8/4
  RES_Brake/1(output1) -> or1/5
  RES_Brake/2(output2) -> or2/5
  RES_Brake/3(output3) -> or3/5
  RES_Brake/4(output4) -> or4/5
  RES_Brake/5(output5) -> or5/5
  RES_Brake/6(output6) -> or6/5
  RES_Brake/7(output7) -> or7/5
  RES_Brake/8(output8) -> or8/5
  RES_ACC/1(output1) -> or1/6
  RES_ACC/2(output2) -> or2/6
  RES_ACC/3(output3) -> or3/6
  RES_ACC/4(output4) -> or4/6
  RES_ACC/5(output5) -> or5/6
  RES_ACC/6(output6) -> or6/6
  RES_ACC/7(output7) -> or7/6
  RES_ACC/8(output8) -> or8/6
  or1/1 -> Conv1/1
  Conv1/1 -> DIAG_RES_INFO_mux/1
  or2/1 -> Conv2/1
  Conv2/1 -> DIAG_RES_INFO_mux/2
  or3/1 -> Conv3/1
  Conv3/1 -> DIAG_RES_INFO_mux/3
  or4/1 -> Conv4/1
  Conv4/1 -> DIAG_RES_INFO_mux/4
  or5/1 -> Conv5/1
  Conv5/1 -> DIAG_RES_INFO_mux/5
  or6/1 -> Conv6/1
  Conv6/1 -> DIAG_RES_INFO_mux/6
  or7/1 -> Conv7/1
  Conv7/1 -> DIAG_RES_INFO_mux/7
  or8/1 -> Conv8/1
  Conv8/1 -> DIAG_RES_INFO_mux/8
  DIAG_RES_INFO_ID/1 -> DIAG_RES_INFO_ID_Out/1
  DIAG_RES_INFO_DLC/1 -> DIAG_RES_INFO_DLC_Out/1
  RES_Steering_in/1 -> RES_Steering/1(RES_Steering)
  RES_Return_INFO_in/1 -> RES_Return_INFO/1(RES_Return_INFO)
  RES_GO_in/1 -> RES_GO/1(RES_GO)
  RES_EBS_in/1 -> RES_EBS/1(RES_EBS)
  RES_Brake_in/1 -> RES_Brake/1(RES_Brake)
  RES_ACC_in/1 -> RES_ACC/1(RES_ACC)

== system FSAC2021_V1_Running/ROUTING/TO_DCAN/Subsystem/DIAG_SCU ==
  Str_Flash_Error_in : Inport
  Str_Encoder_Error_in : Inport  Port=2
  Str_Curr_Error_Fault_in : Inport  Port=3
  Operation_Enabled_in : Inport  Port=4
  Str_UnderVolt_Warning_in : Inport  Port=5
  Str_System_Error_in : Inport  Port=6
  Str_Spd_Over_Alam_in : Inport  Port=7
  Str_PwrMod_TempHigh_Warning_in : Inport  Port=8
  Str_PwrMod_TempHigh_Alarm_in : Inport  Port=9
  Voltage_Enabled_in : Inport  Port=10
  Warning_in : Inport  Port=11
  Str_Para_Error_in : Inport  Port=12
  Str_Overvolt_Warning_in : Inport  Port=13
  Str_Over_TopCurr_in : Inport  Port=14
  Str_Over_SpdError_in : Inport  Port=15
  Str_Over_PosError_in : Inport  Port=16
  Swtiched_On_in : Inport  Port=17
  Str_Limit_Pos_Alarm_in : Inport  Port=18
  Str_I2t_Warning_in : Inport  Port=19
  Str_I2t_Alarm_in : Inport  Port=20
  Fault_in : Inport  Port=21
  Str_Deg_in : Inport  Port=22
  Str_Current_in : Inport  Port=23
  Str_Ang_in : Inport  Port=24
  Conv{1..7} (7 alike) : DataTypeConversion
  DIAG_SCU_mux : Mux  Inputs=7
  Fault : Subsystem
  Operation_Enabled : Subsystem
  Str_Ang : Subsystem
  Str_Curr_Error_Fault : Subsystem
  Str_Current : Subsystem
  Str_Deg : Subsystem
  Str_Encoder_Error : Subsystem
  Str_Flash_Error : Subsystem
  Str_I2t_Alarm : Subsystem
  Str_I2t_Warning : Subsystem
  Str_Limit_Pos_Alarm : Subsystem
  Str_Over_PosError : Subsystem
  Str_Over_SpdError : Subsystem
  Str_Over_TopCurr : Subsystem
  Str_Overvolt_Warning : Subsystem
  Str_Para_Error : Subsystem
  Str_PwrMod_TempHigh_Alarm : Subsystem
  Str_PwrMod_TempHigh_Warning : Subsystem
  Str_Spd_Over_Alam : Subsystem
  Str_System_Error : Subsystem
  Str_UnderVolt_Warning : Subsystem
  Swtiched_On : Subsystem
  Voltage_Enabled : Subsystem
  Warning : Subsystem
  or5 : simulink/Logic and Bit Operations/Bitwise Operator  logicop=OR  UseBitMask=off  NumInputPorts=8  BitMask=bin2dec('11011001')  BitMaskRealWorld=Stored Integer
  or6 : simulink/Logic and Bit Operations/Bitwise Operator  logicop=OR  UseBitMask=off  NumInputPorts=8  BitMask=bin2dec('11011001')  BitMaskRealWorld=Stored Integer
  or7 : simulink/Logic and Bit Operations/Bitwise Operator  logicop=OR  UseBitMask=off  NumInputPorts=5  BitMask=bin2dec('11011001')  BitMaskRealWorld=Stored Integer
  output : Outport
  wires:
  DIAG_SCU_mux/1 -> output/1
  Str_Flash_Error/1(output6) -> or6/1
  Str_Encoder_Error/1(output6) -> or6/2
  Str_Curr_Error_Fault/1(output7) -> or7/3
  Operation_Enabled/1(output5) -> or5/4
  Str_UnderVolt_Warning/1(output6) -> or6/5
  Str_System_Error/1(output5) -> or5/6
  Str_Spd_Over_Alam/1(output7) -> or7/1
  Str_PwrMod_TempHigh_Warning/1(output7) -> or7/4
  Str_PwrMod_TempHigh_Alarm/1(output7) -> or7/2
  Voltage_Enabled/1(output5) -> or5/1
  Warning/1(output5) -> or5/2
  Str_Para_Error/1(output6) -> or6/3
  Str_Overvolt_Warning/1(output6) -> or6/4
  Str_Over_TopCurr/1(output6) -> or6/6
  Str_Over_SpdError/1(output6) -> or6/8
  Str_Over_PosError/1(output7) -> or7/5
  Swtiched_On/1(output5) -> or5/3
  Str_Limit_Pos_Alarm/1(output6) -> or6/7
  Str_I2t_Warning/1(output5) -> or5/5
  Str_I2t_Alarm/1(output5) -> or5/7
  Fault/1(output5) -> or5/8
  Str_Deg/1(output1) -> Conv1/1
  Conv1/1 -> DIAG_SCU_mux/1
  Str_Ang/1(output2) -> Conv2/1
  Conv2/1 -> DIAG_SCU_mux/2
  Str_Ang/2(output3) -> Conv3/1
  Conv3/1 -> DIAG_SCU_mux/3
  Str_Current/1(output4) -> Conv4/1
  Conv4/1 -> DIAG_SCU_mux/4
  or5/1 -> Conv5/1
  Conv5/1 -> DIAG_SCU_mux/5
  or6/1 -> Conv6/1
  Conv6/1 -> DIAG_SCU_mux/6
  or7/1 -> Conv7/1
  Conv7/1 -> DIAG_SCU_mux/7
  Str_Flash_Error_in/1 -> Str_Flash_Error/1(Str_Flash_Error)
  Str_Encoder_Error_in/1 -> Str_Encoder_Error/1(Str_Encoder_Error)
  Str_Curr_Error_Fault_in/1 -> Str_Curr_Error_Fault/1(Str_Curr_Error_Fault)
  Operation_Enabled_in/1 -> Operation_Enabled/1(Operation_Enabled)
  Str_UnderVolt_Warning_in/1 -> Str_UnderVolt_Warning/1(Str_UnderVolt_Warning)
  Str_System_Error_in/1 -> Str_System_Error/1(Str_System_Error)
  Str_Spd_Over_Alam_in/1 -> Str_Spd_Over_Alam/1(Str_Spd_Over_Alam)
  Str_PwrMod_TempHigh_Warning_in/1 -> Str_PwrMod_TempHigh_Warning/1(Str_PwrMod_TempHigh_Warning)
  Str_PwrMod_TempHigh_Alarm_in/1 -> Str_PwrMod_TempHigh_Alarm/1(Str_PwrMod_TempHigh_Alarm)
  Voltage_Enabled_in/1 -> Voltage_Enabled/1(Voltage_Enabled)
  Warning_in/1 -> Warning/1(Warning)
  Str_Para_Error_in/1 -> Str_Para_Error/1(Str_Para_Error)
  Str_Overvolt_Warning_in/1 -> Str_Overvolt_Warning/1(Str_Overvolt_Warning)
  Str_Over_TopCurr_in/1 -> Str_Over_TopCurr/1(Str_Over_TopCurr)
  Str_Over_SpdError_in/1 -> Str_Over_SpdError/1(Str_Over_SpdError)
  Str_Over_PosError_in/1 -> Str_Over_PosError/1(Str_Over_PosError)
  Swtiched_On_in/1 -> Swtiched_On/1(Swtiched_On)
  Str_Limit_Pos_Alarm_in/1 -> Str_Limit_Pos_Alarm/1(Str_Limit_Pos_Alarm)
  Str_I2t_Warning_in/1 -> Str_I2t_Warning/1(Str_I2t_Warning)
  Str_I2t_Alarm_in/1 -> Str_I2t_Alarm/1(Str_I2t_Alarm)
  Fault_in/1 -> Fault/1(Fault)
  Str_Deg_in/1 -> Str_Deg/1(Str_Deg)
  Str_Current_in/1 -> Str_Current/1(Str_Current)
  Str_Ang_in/1 -> Str_Ang/1(Str_Ang)
